simulink model "z5_tran_1"  (R2015a)
settings: Solver=FixedStepDiscrete  StartTime=0.0  StopTime=99.0  FixedStep=1  MaxStep=1  RelTol=1e-3
settings Model: Creator=Bojana Vasic  LastModifiedBy=Bojana Vasic

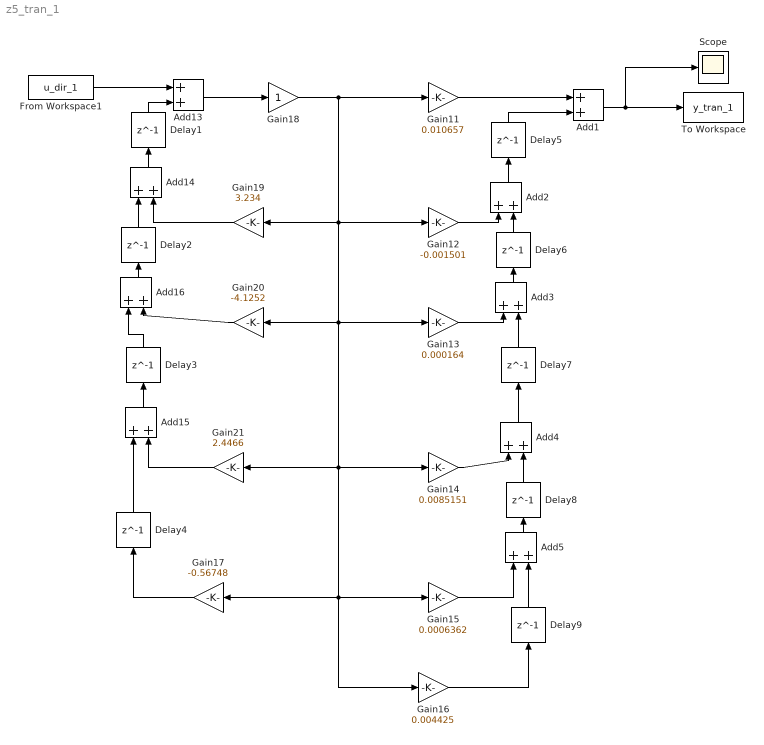
== system z5_tran_1 ==
  Add{1..5,13..16} (9 alike) : Sum
  Delay{1..9} (9 alike) : Delay  DelayLength=1
  From Workspace1 : FromWorkspace  VariableName=u_dir_1  SampleTime=1
  Gain11 : Gain  Gain=0.010657
  Gain12 : Gain  Gain=-0.001501
  Gain13 : Gain  Gain=0.000164
  Gain14 : Gain  Gain=0.0085151
  Gain15 : Gain  Gain=0.0006362
  Gain16 : Gain  Gain=0.004425
  Gain17 : Gain  Gain=-0.56748
  Gain18 : Gain
  Gain19 : Gain  Gain=3.234
  Gain20 : Gain  Gain=-4.1252
  Gain21 : Gain  Gain=2.4466
  Scope : Scope
  To Workspace : ToWorkspace  VariableName=y_tran_1  SampleTime=-1
      settings: Save2DSignal=2-D array (concatenate along first dimension)
  wires:
  Gain18/1 -> Gain12/1, Gain13/1, Gain14/1, Gain16/1, Gain15/1, Gain17/1, Gain21/1, Gain20/1, Gain19/1, Gain11/1
  Add13/1 -> Gain18/1
  From Workspace1/1 -> Add13/1
  Gain11/1 -> Add1/1
  Add1/1 -> Scope/1, To Workspace/1
  Gain19/1 -> Add14/2
  Add14/1 -> Delay1/1
  Delay1/1 -> Add13/2
  Delay2/1 -> Add14/1
  Add16/1 -> Delay2/1
  Gain20/1 -> Add16/2
  Delay3/1 -> Add16/1
  Gain21/1 -> Add15/2
  Add15/1 -> Delay3/1
  Delay4/1 -> Add15/1
  Gain17/1 -> Delay4/1
  Add2/1 -> Delay5/1
  Add3/1 -> Delay6/1
  Add4/1 -> Delay7/1
  Add5/1 -> Delay8/1
  Gain12/1 -> Add2/1
  Delay5/1 -> Add1/2
  Delay6/1 -> Add2/2
  Gain13/1 -> Add3/1
  Delay7/1 -> Add3/2
  Gain14/1 -> Add4/1
  Delay8/1 -> Add4/2
  Gain15/1 -> Add5/1
  Delay9/1 -> Add5/2
  Gain16/1 -> Delay9/1
